simulink model "CT_TOT_nivel"  (Simulink 8.1)
settings: Solver=ode45  StartTime=0.0  StopTime=60  FixedStep=Tm  RelTol=1e-3
InitFcn:
  | Tm = 0.01;
undefined symbols (not defined in the file or in its folder): A, B
libraries: simulink x2
settings Model: Creator=Equipo-Servo  LastModifiedBy=Equipo-Servo  ExtModeTrigDuration=100000
settings DataIOCC: SignalLoggingSaveFormat=Dataset
settings OptimizationCC: ExpressionDepthLimit=128
settings DebuggingCC: FcnCallInpInsideContextMsg=EnableAllAsError
settings HardwareCC: ProdIntDivRoundTo=Zero  ProdEndianess=LittleEndian  ProdHWDeviceType=Generic->32-bit x86 compatible
settings RTWCC: SystemTargetFile=rtwin.tlc  TemplateMakefile=rtwin.tmf  Description=Real-Time Windows Target  ProcessScript=rtwin_make_rtw_hook  RTWCompilerOptimization=On
settings CodeAppCC: MaxIdLength=95
settings RTWinTargetCC: TargetLibSuffix=_rtwin.lib  TargetPreCompLibLocation=C:\Program Files\MATLAB\R2013a\toolbox\rtw\targets\rtwin\lib\win32  CodeReplacementLibrary=ANSI_C  RTWinDir=C:/PROGRA~1/MATLAB/R2013a/toolbox/rtw/targets/rtwin  TargetArch=win32

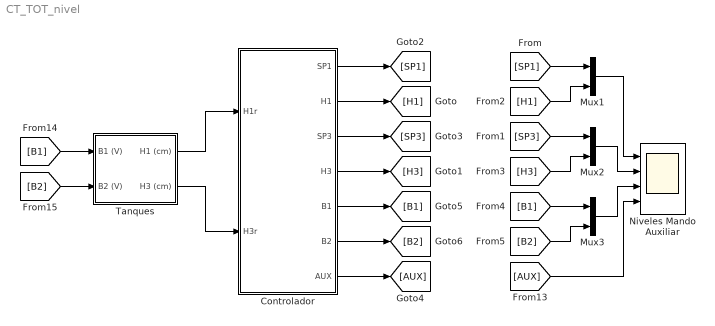
== system CT_TOT_nivel ==
  Controlador : Subsystem
  Mux1 : Mux  Inputs=2
  Mux2 : Mux  Inputs=2
  Mux3 : Mux  Inputs=2
  Niveles Mando Auxiliar : Scope  NumInputPorts=4
      settings: TimeRange=60  YMin=0~-1~0~-5  YMax=15~1~6~15
  Tanques : Subsystem
  wires:
  Mux1/1 -> Niveles Mando Auxiliar/1
  [SP1] -> Mux1/1
  [H1] -> Mux1/2
  [SP3] -> Mux2/1
  [H3] -> Mux2/2
  Mux2/1 -> Niveles Mando Auxiliar/2
  [B1] -> Mux3/1
  [B2] -> Mux3/2
  Mux3/1 -> Niveles Mando Auxiliar/3
  [AUX] -> Niveles Mando Auxiliar/4
  Tanques/1(H1 (cm)) -> Controlador/1(H1r)
  Tanques/2(H3 (cm)) -> Controlador/2(H3r)
  Controlador/1(SP1) -> [SP1]
  Controlador/2(H1) -> [H1]
  Controlador/3(SP3) -> [SP3]
  Controlador/4(H3) -> [H3]
  Controlador/5(B1) -> [B1]
  Controlador/6(B2) -> [B2]
  Controlador/7(AUX) -> [AUX]
  [B1] -> Tanques/1(B1 (V))
  [B2] -> Tanques/2(B2 (V))

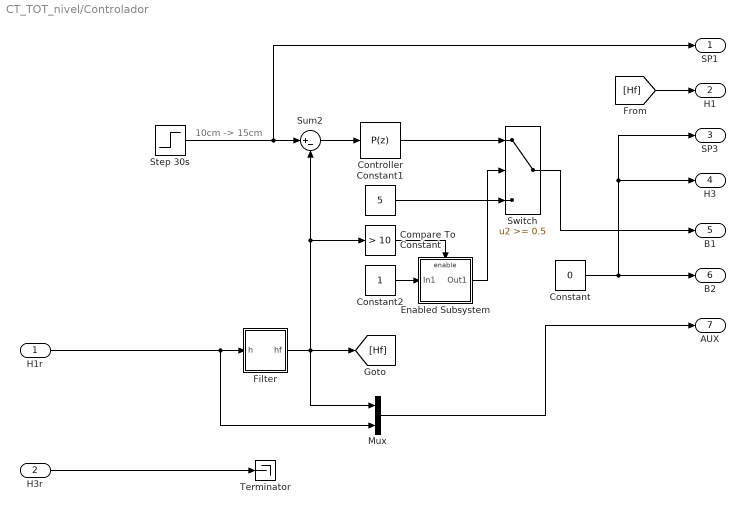
== system CT_TOT_nivel/Controlador ==
  note: 10cm -> 15cm
  H1r : Inport
  H3r : Inport  Port=2
  Compare To Constant : simulink/Logic and Bit Operations/Compare To Constant  relop=>  const=10  OutDataTypeStr=boolean
  Constant : Constant  Value=0
  Constant1 : Constant  Value=5
  Constant2 : Constant
  Controller : simulink/Continuous/PID Controller  Controller=P  TimeDomain=Discrete-time  SampleTime=Tm  IntegratorMethod=Forward Euler  FilterMethod=Forward Euler  Form=Parallel  P=1  I=0  D=0  N=100  InitialConditionSource=internal  InitialConditionForIntegrator=0  InitialConditionForFilter=0  ExternalReset=none  LimitOutput=on  UpperSaturationLimit=5  LowerSaturationLimit=0  LinearizeAsGain=off  AntiWindupMode=back-calculation  Kb=1  TrackingMode=on  Kt=1  PParamMin=[]  PParamMax=[]  IParamMin=[]  IParamMax=[]  DParamMin=[]  DParamMax=[]  NParamMin=[]  NParamMax=[]  KbParamMin=[]  KbParamMax=[]  KtParamMin=[]  KtParamMax=[]  POutMin=[]  POutMax=[]  IOutMin=[]  IOutMax=[]  DOutMin=[]  DOutMax=[]  NOutMin=[]  NOutMax=[]  KbOutMin=[]  KbOutMax=[]  KtOutMin=[]  KtOutMax=[]  IntegratorOutMin=[]  IntegratorOutMax=[]  FilterOutMin=[]  FilterOutMax=[]  SumOutMin=[]  SumOutMax=[]  SumI1OutMin=[]  SumI1OutMax=[]  SumI2OutMin=[]  SumI2OutMax=[]  SumI3OutMin=[]  SumI3OutMax=[]  SumDOutMin=[]  SumDOutMax=[]  SaturationOutMin=[]  SaturationOutMax=[]  IntegratorContinuousStateAttributes=''  IntegratorStateMustResolveToSignalObject=off  IntegratorRTWStateStorageClass=Auto  FilterContinuousStateAttributes=''  FilterStateMustResolveToSignalObject=off  FilterRTWStateStorageClass=Auto
  Enabled Subsystem : Subsystem  TreatAsAtomicUnit=on
  Filter : Subsystem  mask{O=1, Fc=1, Tm=Tm}
      mask prompts: O "Orden"; Fc "Frecuencia de corte"; Tm "Periodo de muestreo"
      mask init:
      | Fm = 1/Tm;
      | [B,A] = butter(O,Fc/(Fm/2));
  Mux : Mux  Inputs=2
  Step 30s : Step  Time=30  Before=10  After=15  SampleTime=0
  Sum2 : Sum  Inputs=|+-
  Switch : Switch  Threshold=0.5
  Terminator : Terminator
  SP1 : Outport
  H1 : Outport  Port=2
  SP3 : Outport  Port=3
  H3 : Outport  Port=4
  B1 : Outport  Port=5
  B2 : Outport  Port=6
  AUX : Outport  Port=7
  wires:
  Step 30s/1 -> SP1/1, Sum2/1
  H1r/1 -> Mux/2, Filter/1(h)
  Filter/1(hf) -> [Hf], Mux/1, Compare To Constant/1, Sum2/2
  Mux/1 -> AUX/1
  H3r/1 -> Terminator/1
  Constant/1 -> SP3/1, H3/1, B2/1
  Controller/1 -> Switch/1
  Constant1/1 -> Switch/3
  Compare To Constant/1 -> Enabled Subsystem/Enable
  Constant2/1 -> Enabled Subsystem/1(In1)
  Sum2/1 -> Controller/1
  Switch/1 -> B1/1
  [Hf] -> H1/1
  Enabled Subsystem/1(Out1) -> Switch/2

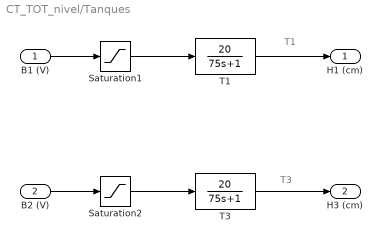
== system CT_TOT_nivel/Tanques ==
  note: T3
  note: T1
  B1 (V) : Inport
  B2 (V) : Inport  Port=2
  Saturation1 : Saturate  UpperLimit=5  LowerLimit=0
  Saturation2 : Saturate  UpperLimit=5  LowerLimit=0
  T1 : TransferFcn  Numerator=[20]  Denominator=[75 1]
  T3 : TransferFcn  Numerator=[20]  Denominator=[75 1]
  H1 (cm) : Outport
  H3 (cm) : Outport  Port=2
  wires:
  T1/1 -> H1 (cm)/1
  B1 (V)/1 -> Saturation1/1
  Saturation1/1 -> T1/1
  B2 (V)/1 -> Saturation2/1
  Saturation2/1 -> T3/1
  T3/1 -> H3 (cm)/1

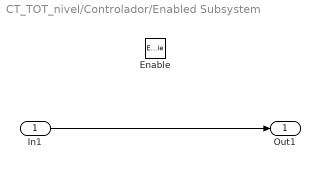
== system CT_TOT_nivel/Controlador/Enabled Subsystem ==
  In1 : Inport
  Enable : EnablePort
  Out1 : Outport
  wires:
  In1/1 -> Out1/1

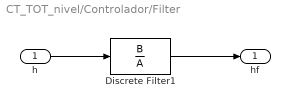
== system CT_TOT_nivel/Controlador/Filter ==
  h : Inport
  Discrete Filter1 : DiscreteFilter  Numerator=B  Denominator=A  SampleTime=Tm
  hf : Outport
  wires:
  Discrete Filter1/1 -> hf/1
  h/1 -> Discrete Filter1/1
